simulink model "INVERTOR_IN_MATLAB_SING_MOSFET"  (R2018a)
settings: Solver=VariableStepAuto  StartTime=0.0  StopTime=10.0  RelTol=1e-3
libraries: powerlib x14, powerlib_meascontrol x1
settings Model: Creator=pursh  LastModifiedBy=pursh

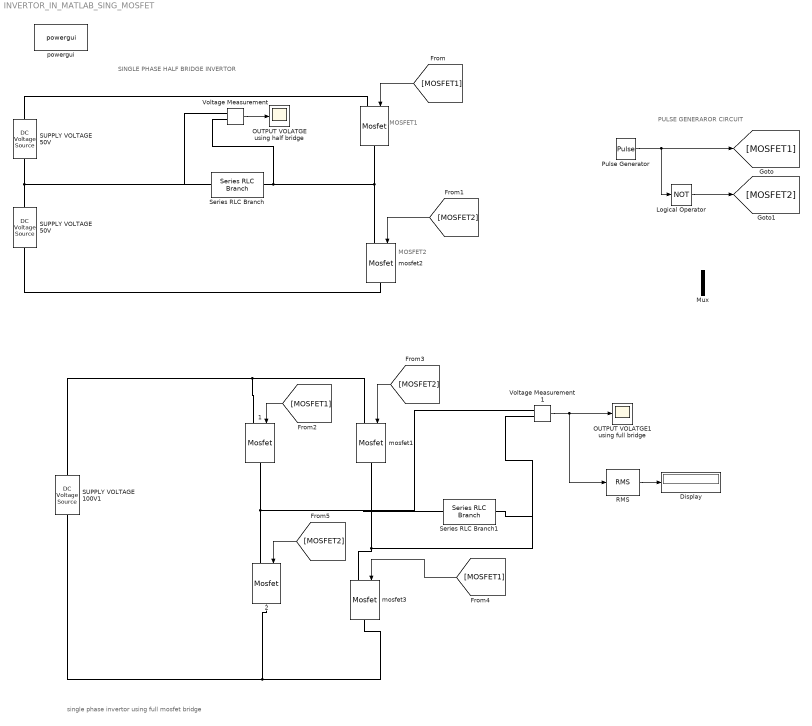
== system INVERTOR_IN_MATLAB_SING_MOSFET ==
  note: single phase invertor using full mosfet bridge
  note: SINGLE PHASE HALF BRIDGE INVERTOR
  note: PULSE GENERAROR CIRCUIT
  note: MOSFET2
  note: MOSFET1
  " " : powerlib/Power Electronics/Mosfet  Ron=0.1  Lon=0  Rd=0.01  Vfd=0  IC=0  Rs=1e5  Cs=inf  Measurements=off
  " 1" : powerlib/Power Electronics/Mosfet  Ron=0.1  Lon=0  Rd=0.01  Vfd=0  IC=0  Rs=1e5  Cs=inf  Measurements=off
  " 2" : powerlib/Power Electronics/Mosfet  Ron=0.1  Lon=0  Rd=0.01  Vfd=0  IC=0  Rs=1e5  Cs=inf  Measurements=off
  Display : Display
  Logical Operator : Logic  Operator=NOT  AllPortsSameDT=off  OutDataTypeStr=boolean
  Mux : Mux  Inputs=2
  OUTPUT VOLATGE using half bridge : Scope
  "OUTPUT VOLATGE1 using full bridge " : Scope
  Pulse Generator : DiscretePulseGenerator  PulseType=Time based  Period=2e-5  PulseWidth=50
  RMS : powerlib_meascontrol/Measurements/RMS  TrueRMS=on  Freq=60  RMSInit=120  Ts=0
  SUPPLY VOLTAGE 100V1 : powerlib/Electrical Sources/DC Voltage Source  Amplitude=100  Measurements=None
  SUPPLY VOLTAGE 50V : powerlib/Electrical Sources/DC Voltage Source  Amplitude=50  Measurements=None
  "SUPPLY VOLTAGE 50V " : powerlib/Electrical Sources/DC Voltage Source  Amplitude=50  Measurements=None
  Series RLC Branch : powerlib/Elements/Series RLC Branch  LConnTagsString=__new0  RConnTagsString=__new0  BranchType=R  Resistance=50  Inductance=1e-3  SetiL0=off  InitialCurrent=0  Capacitance=1e-6  Setx0=off  InitialVoltage=0  Measurements=None
  Series RLC Branch1 : powerlib/Elements/Series RLC Branch  LConnTagsString=__new0  RConnTagsString=__new0  BranchType=R  Resistance=50  Inductance=1e-3  SetiL0=off  InitialCurrent=0  Capacitance=1e-6  Setx0=off  InitialVoltage=0  Measurements=None
  Voltage Measurement : powerlib/Measurements/Voltage Measurement  PhasorSimulation=off  OutputType=Complex  PSBequivalent=0
  Voltage Measurement1 : powerlib/Measurements/Voltage Measurement  PhasorSimulation=off  OutputType=Complex  PSBequivalent=0
  mosfet1 : powerlib/Power Electronics/Mosfet  Ron=0.1  Lon=0  Rd=0.01  Vfd=0  IC=0  Rs=1e5  Cs=inf  Measurements=off
  mosfet2 : powerlib/Power Electronics/Mosfet  Ron=0.1  Lon=0  Rd=0.01  Vfd=0  IC=0  Rs=1e5  Cs=inf  Measurements=off
  mosfet3 : powerlib/Power Electronics/Mosfet  Ron=0.1  Lon=0  Rd=0.01  Vfd=0  IC=0  Rs=1e5  Cs=inf  Measurements=off
  powergui : powerlib/powergui  Priority=1  SimulationMode=Continuous  SampleTime=50e-6  frequency=60  Iterations=50  frequencyindice=0  Pbase=100e6  ErrMax=1e-4  UnitsV=kV  UnitsW=MW  buscounter=0  FunctionMessages=off  echomessages=off  EnableUseOfTLC=off  CurrentSourceSwitches=off  DisableSnubberDevices=off  DisableRonSwitches=off  DisableVfSwitches=off  DisplayEquations=off  SolverType=Tustin/Backward Euler (TBE)  Interpol=off  ExternalGateDelay=off  methode=off  Ts=100  x0status=blocks  SPID=on  SwTol=0  HookPort=off  RestoreLinks=warning  ResistiveCurrentMeasurement=off  Frange=[0:2:500]  Ylog=off  Xlog=on  ShowGrid=off  save=off  variable=ZData  structure=0  ZoomFFT=off  StartTime=0.0  cycles=1  DisplayStyle=1  fundamental=60  FreqAxis=off  MaxFrequency=1000  frequencyindicesteady=1  RmsSteady=1  display=off
  wires:
  Voltage Measurement/1 -> OUTPUT VOLATGE using half bridge/1
  Pulse Generator/1 -> Logical Operator/1, [MOSFET1]
  Logical Operator/1 -> [MOSFET2]
  [MOSFET1] -> " "/1
  [MOSFET2] -> mosfet2/1
  Voltage Measurement1/1 -> RMS/1, "OUTPUT VOLATGE1 using full bridge "/1
  [MOSFET2] -> " 2"/1
  [MOSFET1] -> mosfet3/1
  [MOSFET2] -> mosfet1/1
  [MOSFET1] -> " 1"/1
  RMS/1 -> Display/1
  connections:
  SUPPLY VOLTAGE 50V/RConn1 -- " "/LConn1
  "SUPPLY VOLTAGE 50V "/LConn1 -- mosfet2/RConn1
  "SUPPLY VOLTAGE 50V "/RConn1 -- Voltage Measurement/LConn1 -- Series RLC Branch/LConn1 -- SUPPLY VOLTAGE 50V/LConn1
  Series RLC Branch/RConn1 -- Voltage Measurement/LConn2 -- " "/RConn1 -- mosfet2/LConn1
  SUPPLY VOLTAGE 100V1/RConn1 -- " 1"/LConn1 -- mosfet1/LConn1
  " 1"/RConn1 -- Voltage Measurement1/LConn1 -- Series RLC Branch1/LConn1 -- " 2"/LConn1
  mosfet1/RConn1 -- Series RLC Branch1/RConn1 -- Voltage Measurement1/LConn2 -- mosfet3/LConn1
  SUPPLY VOLTAGE 100V1/LConn1 -- " 2"/RConn1 -- mosfet3/RConn1
